simulink model "Three_Phase_Buck_Converter"  (R2023b)
settings: Solver=ode45  StartTime=0.0  StopTime=0.001  MaxStep=1e-06  RelTol=1e-3  EnableMultiTasking=on
libraries: simulink x7, spsMosfetLib x6, spsCurrentMeasurementLib x5, spsSeriesRLCBranchLib x5, spsDCVoltageSourceLib x1, spsVoltageMeasurementLib x1, sps_lib x1
settings Model: Creator=Karuna  LastModifiedBy=HP
settings SolverCC: AlgebraicLoopSolver=TrustRegion
settings DataIOCC: LimitDataPoints=on  SaveFormat=Array  SignalLoggingSaveFormat=ModelDataLogs  ReturnWorkspaceOutputs=off
settings OptimizationCC: ExpressionDepthLimit=2147483647  LifeSpan=inf
settings DebuggingCC: UnderspecifiedInitializationDetection=Classic  MergeDetectMultiDrivingBlocksExec=none  SolverPrmCheckMsg=warning  FcnCallInpInsideContextMsg=warning  UnconnectedInputMsg=warning  UnconnectedOutputMsg=warning  UnconnectedLineMsg=warning  StateNameClashWarn=warning  SFUnexpectedBacktrackingDiag=warning  SFNoUnconditionalDefaultTransitionDiag=warning  SFExecutionAtInitializationDiag=none  ArithmeticOperatorsInVariantConditions=warning
settings HardwareCC: ProdBitPerPointer=32  ProdBitPerSizeT=32  ProdBitPerPtrDiffT=32  ProdLargestAtomicFloat=None  ProdIntDivRoundTo=Undefined  ProdEndianess=Unspecified  ProdWordSize=32  ProdHWDeviceType=32-bit Generic
settings ModelReferenceCC: PropagateSignalLabelsOutOfModel=off
settings SFSimCC: SimUseLocalCustomCode=off  CustomCodeUndefinedFunction=UseInterfaceOnly
settings RTWCC: RTWUseLocalCustomCode=off
settings CodeAppCC: StateflowObjectComments=on
settings GRTTargetCC: TargetLangStandard=C89/C90 (ANSI)  CombineOutputUpdateFcns=off  GRTInterface=on
settings ConfigComp: CovMetricSettings=dw  CovSaveCumulativeToWorkspaceVar=on  CovSaveSingleToWorkspaceVar=on  CovExternalEMLEnable=off

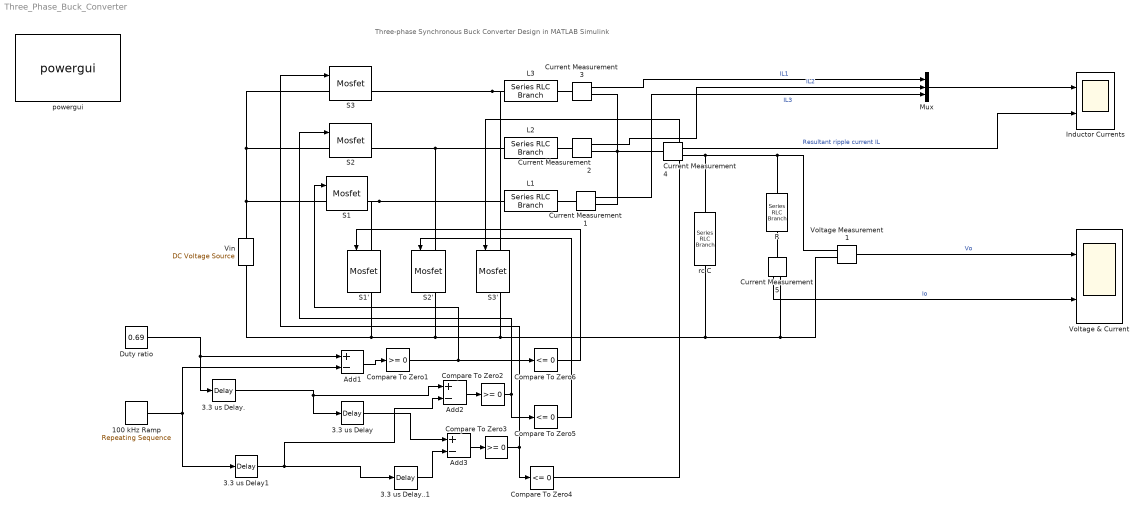
== system Three_Phase_Buck_Converter ==
  note: Three-phase Synchronous Buck Converter Design in MATLAB Simulink
  100 kHz Ramp : simulink/Sources/Repeating Sequence  rep_seq_t=[0 10e-06]  rep_seq_y=[0 1]
  3.3 us Delay. : TransportDelay  DelayTime=3.3333e-06
  "3.3 us Delay " : TransportDelay  DelayTime=3.3333e-06
  3.3 us Delay..1 : TransportDelay  DelayTime=3.3333e-06
  3.3 us Delay1 : TransportDelay  DelayTime=3.3333e-06
  Add1 : Sum  Inputs=+-
  Add2 : Sum  Inputs=+-
  Add3 : Sum  Inputs=+-
  Compare To Zero1 : simulink/Logic and Bit Operations/Compare To Zero  relop=>=  OutDataTypeStr=uint8
  Compare To Zero2 : simulink/Logic and Bit Operations/Compare To Zero  relop=>=  OutDataTypeStr=uint8
  Compare To Zero3 : simulink/Logic and Bit Operations/Compare To Zero  relop=>=  OutDataTypeStr=uint8
  Compare To Zero4 : simulink/Logic and Bit Operations/Compare To Zero  relop=<=  OutDataTypeStr=uint8
  Compare To Zero5 : simulink/Logic and Bit Operations/Compare To Zero  relop=<=  OutDataTypeStr=uint8
  Compare To Zero6 : simulink/Logic and Bit Operations/Compare To Zero  relop=<=  OutDataTypeStr=uint8
  Current Measurement{1..5} (5 alike) : spsCurrentMeasurementLib/Current Measurement  PhasorSimulation=off  OutputType=Complex  PSBequivalent=0
  Duty ratio : Constant  Value=0.69
  Inductor Currents : Scope  NumInputPorts=2
  L1 : spsSeriesRLCBranchLib/Series RLC Branch  LConnTagsString=__new0  RConnTagsString=__new0  BranchType=L  Resistance=1  Inductance=2.1723e-005  SetiL0=off  InitialCurrent=0  Capacitance=1e-6  Setx0=off  InitialVoltage=0  Measurements=None
  L2 : spsSeriesRLCBranchLib/Series RLC Branch  LConnTagsString=__new0  RConnTagsString=__new0  BranchType=L  Resistance=1  Inductance=2.1723e-005  SetiL0=off  InitialCurrent=0  Capacitance=1e-6  Setx0=off  InitialVoltage=0  Measurements=None
  L3 : spsSeriesRLCBranchLib/Series RLC Branch  LConnTagsString=__new0  RConnTagsString=__new0  BranchType=L  Resistance=1  Inductance=2.1723e-005  SetiL0=off  InitialCurrent=0  Capacitance=1e-6  Setx0=off  InitialVoltage=0  Measurements=None
  Mux : Mux  Inputs=3
  R : spsSeriesRLCBranchLib/Series RLC Branch  LConnTagsString=__new0  RConnTagsString=__new0  BranchType=R  Resistance=1.1520  Inductance=1e-3  SetiL0=off  InitialCurrent=0  Capacitance=1e-6  Setx0=off  InitialVoltage=0  Measurements=None
  S1 : spsMosfetLib/Mosfet  Ron=0.02  Lon=0  Rd=0.001  Vfd=0  IC=0  Rs=1e5  Cs=inf  Measurements=on
  S1' : spsMosfetLib/Mosfet  Ron=0.02  Lon=0  Rd=0.001  Vfd=0  IC=0  Rs=1e5  Cs=inf  Measurements=on
  S2 : spsMosfetLib/Mosfet  Ron=0.02  Lon=0  Rd=0.001  Vfd=0  IC=0  Rs=1e5  Cs=inf  Measurements=on
  S2' : spsMosfetLib/Mosfet  Ron=0.02  Lon=0  Rd=0.001  Vfd=0  IC=0  Rs=1e5  Cs=inf  Measurements=on
  S3 : spsMosfetLib/Mosfet  Ron=0.02  Lon=0  Rd=0.001  Vfd=0  IC=0  Rs=1e5  Cs=inf  Measurements=on
  S3' : spsMosfetLib/Mosfet  Ron=0.02  Lon=0  Rd=0.001  Vfd=0  IC=0  Rs=1e5  Cs=inf  Measurements=on
  Vin : spsDCVoltageSourceLib/DC Voltage Source  Amplitude=35  Measurements=None
  Voltage & Current : Scope  NumInputPorts=2
  Voltage Measurement1 : spsVoltageMeasurementLib/Voltage Measurement  PhasorSimulation=off  OutputType=Complex  PSBequivalent=0
  powergui : sps_lib/powergui  Priority=1  SimulationMode=Continuous  SampleTime=50e-6  frequency=60  Iterations=50  frequencyindice=0  Pbase=100e6  ErrMax=1e-4  UnitsV=kV  UnitsW=MW  buscounter=0  FunctionMessages=off  echomessages=off  EnableUseOfTLC=off  CurrentSourceSwitches=on  DisableSnubberDevices=off  DisableRonSwitches=off  DisableVfSwitches=off  DisplayEquations=off  AutomaticDiscreteSolvers=off  SolverType=Tustin/Backward Euler (TBE)  Interpol=off  ExternalGateDelay=off  methode=off  Ts=100  x0status=blocks  SPID=off  SwTol=0  HookPort=off  NonlinearTolerance=1e-4  nMaxIteration=100  ContinueOnMaxIteration=off  RestoreLinks=warning  ResistiveCurrentMeasurement=off  Frange=[0:2:500]  Ylog=off  Xlog=on  ShowGrid=off  save=off  variable=ZData  structure=0  ZoomFFT=off  StartTime=0.0  cycles=1  DisplayStyle=1  fundamental=60  FreqAxis=off  MaxFrequency=1000  frequencyindicesteady=1  RmsSteady=1  display=off
  rc C : spsSeriesRLCBranchLib/Series RLC Branch  LConnTagsString=__new0  RConnTagsString=__new0  BranchType=RC  Resistance=0.01  Inductance=1e-3  SetiL0=off  InitialCurrent=0  Capacitance=3.3e-06  Setx0=off  InitialVoltage=0  Measurements=None
  wires:
  3.3 us Delay./1 -> Add2/1, "3.3 us Delay "/1
  3.3 us Delay1/1 -> 3.3 us Delay..1/1, Add2/2
  "3.3 us Delay "/1 -> Add3/1
  3.3 us Delay..1/1 -> Add3/2
  Add3/1 -> Compare To Zero3/1
  Add2/1 -> Compare To Zero2/1
  Add1/1 -> Compare To Zero1/1
  Compare To Zero1/1 -> S1/1, Compare To Zero6/1
  Compare To Zero2/1 -> Compare To Zero5/1, S2/1
  Compare To Zero3/1 -> Compare To Zero4/1, S3/1
  Compare To Zero6/1 -> S1'/1
  Compare To Zero4/1 -> S3'/1
  Duty ratio/1 -> Add1/1, 3.3 us Delay./1
  Compare To Zero5/1 -> S2'/1
  Voltage Measurement1/1 -> Voltage & Current/1  "Vo"
  Current Measurement5/1 -> Voltage & Current/2  "Io"
  Current Measurement3/1 -> Mux/1  "IL1"
  Current Measurement2/1 -> Mux/2  "IL2"
  Mux/1 -> Inductor Currents/1
  Current Measurement1/1 -> Mux/3  "IL3"
  Current Measurement4/1 -> Inductor Currents/2  "Resultant ripple current IL"
  100 kHz Ramp/1 -> Add1/2, 3.3 us Delay1/1
  connections:
  S1'/LConn1 -- L1/LConn1 -- S1/RConn1
  S2'/LConn1 -- L2/LConn1 -- S2/RConn1
  S3'/LConn1 -- S3/RConn1 -- L3/LConn1
  Current Measurement2/RConn1 -- Current Measurement4/LConn1 -- Current Measurement3/RConn1 -- Current Measurement1/RConn1
  Vin/LConn1 -- S1'/RConn1 -- S2'/RConn1 -- S3'/RConn1 -- Current Measurement5/RConn1 -- Voltage Measurement1/LConn2 -- rc C/RConn1
  rc C/LConn1 -- Current Measurement4/RConn1 -- R/LConn1 -- Voltage Measurement1/LConn1
  Vin/RConn1 -- S2/LConn1 -- S3/LConn1 -- S1/LConn1
  Current Measurement5/LConn1 -- R/RConn1
  L2/RConn1 -- Current Measurement2/LConn1
  Current Measurement3/LConn1 -- L3/RConn1
  Current Measurement1/LConn1 -- L1/RConn1
